simulink model "lab3task1"  (R2021a)
settings: Solver=VariableStepAuto  StartTime=0.0  StopTime=10.0  RelTol=1e-3
libraries: simulink x2
settings Model: Creator=youssefashraf  LastModifiedBy=youssefashraf

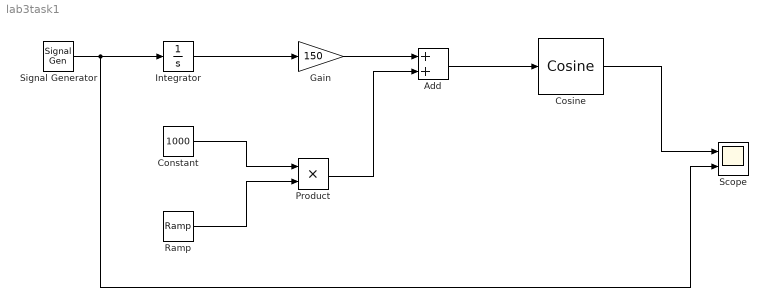
== system lab3task1 ==
  Add : Sum
  Constant : Constant  Value=1000
  Cosine : simulink/Lookup Tables/Cosine  Formula=cos(2*pi*u)  NumDataPoints=(2^5)+1  OutputWordLength=16  InternalRulePriority=Speed
      settings: SourceProductBaseCode=SL
  Gain : Gain  Gain=150
  Integrator : Integrator
  Product : Product
  Ramp : simulink/Sources/Ramp  slope=1  start=0  InitialOutput=0
  Scope : Scope  NumInputPorts=2
  Signal Generator : SignalGenerator  Amplitude=2  Frequency=100
  wires:
  Signal Generator/1 -> Scope/2, Integrator/1
  Integrator/1 -> Gain/1
  Gain/1 -> Add/1
  Constant/1 -> Product/1
  Ramp/1 -> Product/2
  Product/1 -> Add/2
  Add/1 -> Cosine/1
  Cosine/1 -> Scope/1
